simulink library "lib_Solver"  (R2021a)
settings: Solver=VariableStepAuto  StartTime=0.0  StopTime=10.0  RelTol=1e-3
settings Model: Creator=chiar  LastModifiedBy=chiar

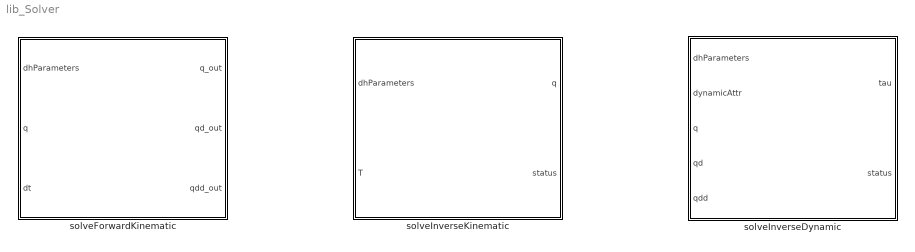
== system lib_Solver ==
  solveForwardKinematic : MATLAB Function  TreatAsAtomicUnit=on
  solveInverseDynamic : MATLAB Function  TreatAsAtomicUnit=on
  solveInverseKinematic : MATLAB Function  TreatAsAtomicUnit=on

== matlab function lib_Solver/solveInverseKinematic ==
  data: dhParameters input; T input; q output; status output
function [q, status] = solveInverseKinematics(dhParameters, T)
dim = size(T);
if (dim(1) == 3 && dim(2) == 1) || ...
        (dim(1) == 1 && dim(2) == 3)
    % define homogeneous transform T from pose
    TT = [1, 0, 0, T(1, 1);
        0, -1, 0, T(2, 1);
        0, 0, -1, T(3, 1);
        0, 0, 0, 1];
else 
    TT = T;
end
dhParams = struct2table(dhParameters);
[q, status] = solver.solveInverseKinematics(dhParams, TT);
end

== matlab function lib_Solver/solveInverseDynamic ==
  data: dhParameters input; dynamicAttr input; q input; tau output; qd input; qdd input; status output
function [tau, status] = solveInverseDynamic(dhParameters, dynamicAttr, q, qd, qdd)

dhParams = struct2table(dhParameters);
[tau, status] = solver.solveInverseDynamic(dhParams, ...
    dynamicAttr.M, ...
    dynamicAttr.I, ...
    dynamicAttr.Fext, ...
    q, qd, qdd);

end

== matlab function lib_Solver/solveForwardKinematic ==
  data: dhParameters input; q input; q_out output; qd_out output; dt input; qdd_out output
function [q_out, qd_out, qdd_out] = solveForwardKinematics(dhParameters, q, dt)
coder.internal.errorIf(nargin > 2 & nargout < 3, 'solver:solveForwardKinematics:NotEnoughInputArgument');
dhParams = struct2table(dhParameters);
[q_out, qd_out, qdd_out] = solver.solveForwardKinematics(dhParams, q, dt);
end
